simulink library "Lib_Vol_PropLookup_TMATS"  (R2015a)
settings: Solver=ode45  StartTime=0.0  StopTime=10.0  RelTol=1e-3
undefined symbols (not defined in the file or in its folder): hP_PropArray_M, htVec_M, PtVec_M, sP_PropArray_M, sVec_M, TtVec_M
Description:
  | Thomas Modules
settings Model: Creator=jwchapm2  LastModifiedBy=jwchapm2
settings OptimizationCC: ExpressionDepthLimit=2147483647
settings DebuggingCC: UnderspecifiedInitializationDetection=Classic  MergeDetectMultiDrivingBlocksExec=none  SolverPrmCheckMsg=warning  StateNameClashWarn=warning

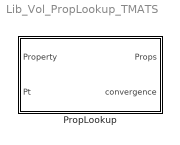
== system Lib_Vol_PropLookup_TMATS ==
  PropLookup : Subsystem  TreatAsAtomicUnit=on  mask(T-MATS: PropLookup Library Block){case_M='ht', propg_M=0, htg_M=0, htVec_M=[0 10], PtVec_M=[0 10], TtVec_M=[0 10], sVec_M=[0 10], htArray_M=ones(length(TtVec_M), length(PtVec_M)), rhoArray_M=ones(length(htVec_M), length(PtVec_M)), uArray_M=ones(length(htVec_M), length(PtVec_M)), sArray_M=ones(length(htVec_M), length(PtVec_M)), muArray_M=ones(length(htVec_M), length(PtVec_M)), ThArray_M=ones(length(htVec_M), length(PtVec_M)), CvArray_M=ones(length(htVec_M), length(PtVec_M)), CpArray_M=ones(length(htVec_M), length(PtVec_M)), kArray_M=ones(length(htVec_M), length(PtVec_M)), TsArray_M=ones(length(sVec_M), length(PtVec_M)), hsArray_M=ones(length(sVec_M), length(PtVec_M)), Rval_M=0}
      mask prompts: case_M "case_M - Property type"; propg_M "propg_M - Initial guess for property value"; htg_M "htg_M - Initial guess for ethanply value"; htVec_M "htVec_M - ht axis for table lookup"; PtVec_M "PtVec_M - Pt axis for table lookup"; TtVec_M "TtVec_M - Tt axis for table lookup"; sVec_M "sVec_M - s axis for table lookup"; htArray_M "htArray_M - enthlapy Array f(Tt,Pt)"; rhoArray_M "rhoArray_M - rho Array f(ht,Pt)"; uArray_M "uArray_M - u Array f(ht,Pt)"; sArray_M "sArray_M - s Array f(ht,Pt)"; muArray_M "muArray_M - mu Array f(ht,Pt)"; ThArray_M "ThArray_M - Th Array f(ht,Pt)"; CvArray_M "CvArray_M - Cv Array f(ht,Pt)"; CpArray_M "CpArray_M - Cp Array f(ht,Pt)"; kArray_M "kArray_M - k Array f(ht,Pt)"; TsArray_M "TsArray_M - Ts Array f(s,Pt)"; hsArray_M "hsArray_M - hs Array f(s,Pt)"; Rval_M "Rval_M - R value"
      mask help: This block is used to model the thermodynamic properties of a mass flow based on table lookups.
      mask init:
      | hP_PropArray_M(:,:,1) = rhoArray_M;
      | hP_PropArray_M(:,:,2) = uArray_M;
      | hP_PropArray_M(:,:,3) = sArray_M;
      | hP_PropArray_M(:,:,4) = muArray_M;
      | hP_PropArray_M(:,:,5) = ThArray_M;
      | hP_PropArray_M(:,:,6) = CvArray_M;
      | hP_PropArray_M(:,:,7) = kArray_M;
      | hP_PropArray_M(:,:,8) = CpArray_M;
      | 
      | sP_PropArray_M(:,:,1) = TsArray_M;
      | sP_PropArray_M(:,:,2) = hsArray_M;
      | 
      | case_M = double(case_M);
      mask Help: web(which('Vol_TMATS_PropLookup.html'),'-helpbrowser')

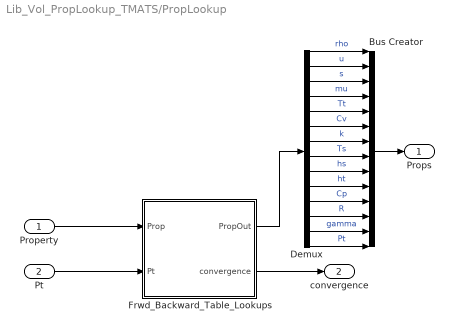
== system Lib_Vol_PropLookup_TMATS/PropLookup ==
  Property : Inport
  Pt : Inport  Port=2
  Bus Creator : BusCreator  Inputs=14
  Demux : Demux  Outputs=14
  Frwd_Backward_Table_Lookups : MATLAB Function  TreatAsAtomicUnit=on
  Props : Outport
  convergence : Outport  Port=2
  wires:
  Property/1 -> Frwd_Backward_Table_Lookups/1(Prop)
  Pt/1 -> Frwd_Backward_Table_Lookups/2(Pt)
  Frwd_Backward_Table_Lookups/2(convergence) -> convergence/1
  Demux/13 -> Bus Creator/13  "gamma"
  Demux/12 -> Bus Creator/12  "R"
  Demux/11 -> Bus Creator/11  "Cp"
  Demux/10 -> Bus Creator/10  "ht"
  Demux/8 -> Bus Creator/8  "Ts"
  Demux/7 -> Bus Creator/7  "k"
  Demux/4 -> Bus Creator/4  "mu"
  Demux/9 -> Bus Creator/9  "hs"
  Demux/6 -> Bus Creator/6  "Cv"
  Demux/3 -> Bus Creator/3  "s"
  Demux/5 -> Bus Creator/5  "Tt"
  Demux/2 -> Bus Creator/2  "u"
  Demux/1 -> Bus Creator/1  "rho"
  Bus Creator/1 -> Props/1
  Frwd_Backward_Table_Lookups/1(PropOut) -> Demux/1
  Demux/14 -> Bus Creator/14  "Pt"

== matlab function Lib_Vol_PropLookup_TMATS/PropLookup/Frwd_Backward_Table_Lookups ==
  data: Prop input; Pt input; PropOut output; convergence output; htg_M parameter; htVec_M parameter; TtVec_M parameter; PtVec_M parameter; sVec_M parameter; htArray_M parameter; hP_PropArray_M parameter; sP_PropArray_M parameter; Rval_M parameter; case_M parameter
function [PropOut, convergence] = fcn(Prop, Pt, htg_M, htVec_M, TtVec_M, PtVec_M, sVec_M, htArray_M, hP_PropArray_M, sP_PropArray_M, Rval_M, case_M)
% Table lookup based on ht or ht guess

%gather table vector table data
htVec = htVec_M;
TtVec = TtVec_M;
PtVec = PtVec_M;
sVec = sVec_M;

% determine min and max table lookup values
Tmx = max(TtVec);
Tmn = min(TtVec);
hmx = max(htVec);
hmn = min(htVec);
Pmx = max(PtVec);
Pmn = min(PtVec);
smx = max(sVec);
smn = min(sVec);

Pt_tbl = max(min(Pt,Pmx),Pmn);

%gather table array data
rhoArray    =  hP_PropArray_M(:,:,1);
uArray      =  hP_PropArray_M(:,:,2);
sArray      =  hP_PropArray_M(:,:,3);
muArray     =  hP_PropArray_M(:,:,4);
ThArray     =  hP_PropArray_M(:,:,5);
CvArray     =  hP_PropArray_M(:,:,6);
kArray      =  hP_PropArray_M(:,:,7);
CpArray     =  hP_PropArray_M(:,:,8);


TsArray = sP_PropArray_M(:,:,1);
hsArray = sP_PropArray_M(:,:,2);

htArray = htArray_M;


switch char(case_M)
    case 'ht'
        iterate = 0;
        htg = Prop;
    case 'Tt'
        iterate = 0;
        T_tbl = max(min(Prop,Tmx),Tmn);
        htg = interp2(TtVec, PtVec, htArray,T_tbl, Pt_tbl);
    otherwise
        iterate = 1;
end

iter = 0;
maxiter = 15 ;

if iterate == 1 % ht is unknown,  iterate to find it based on what Prop is
    
    % determine initial error, ht guess term, and iteration constants
    switch char(case_M)
        case 'u'
            itprop = interp2(htVec, PtVec, rhoArray,htg_M, Pt);
        case 's'
            itprop = interp2(htVec, PtVec, sArray,htg_M, Pt);
        case 'k'
            itprop = interp2(htVec, PtVec, kArray,htg_M, Pt);
        case 'Ts'
            s_prop = interp2(htVec, PtVec, sArray,htg_M, Pt);
            itprop = interp2(sVec, PtVec, TsArray,s_prop, Pt);
        case 'hs'
            s_prop = interp2(htVec, PtVec, sArray,htg_M, Pt);
            itprop = interp2(sVec, PtVec, hsArray, s_prop, Pt);
        otherwise
            itprop = 0;
    end
    Error = Prop - itprop;
    htg_new = htg_M + 0.002;
    erthr = 0.0001;
    htg = htg_M;
    
    while ((abs(Error) > erthr) && (iter < maxiter))
        % Set old values before recaulcation
        Er_old = Error;
        htg_old = htg;
        
        % if step is too low assume larger step
        if abs(htg - htg_new) < 0.001
            htg = htg + 0.002;
        else
            htg = htg_new;
        end
        
        htg_tbl = max(min(htg,hmx),hmn);
        
        % Determine property term based on guessed ht
        switch char(case_M)
            case 'u'
                itprop = interp2(htVec, PtVec, rhoArray,htg_tbl, Pt_tbl);
            case 's'
                itprop = interp2(htVec, PtVec, sArray,htg_tbl, Pt_tbl);
            case 'k'
                itprop = interp2(htVec, PtVec, kArray,htg_tbl, Pt_tbl);
            case 'Ts'
                s_prop = interp2(htVec, PtVec, sArray,htg_tbl, Pt_tbl);
                s_ptbl = max(min(s_prop,smx),smn);
                itprop = interp2(sVec, PtVec, TsArray,s_ptbl, Pt_tbl);
            case 'hs'
                s_prop = interp2(htVec, PtVec, sArray,htg_tbl, Pt_tbl);
                s_ptbl = max(min(s_prop,smx),smn);
                itprop = interp2(sVec, PtVec, hsArray, s_ptbl, Pt_tbl);
            otherwise
                itprop = 0;
        end
        % determine current property term error
        Error = Prop - itprop;
        
        if (abs(Error) > erthr)
            % determine new guess enthalpy by secant algorithm
            htg_new = htg - Error *(htg - htg_old)/(Error - Er_old);
        end
        iter = iter +1;
    end
end

if iter >= maxiter
    convergence = 0;
else
    convergence = 1;
end

%generate outputs based on ht (found by input, table lookup, or iteration)
ht = htg;

ht_tbl = max(min(ht,hmx),hmn);

% ht, Pt generated lookups
rho = interp2(htVec, PtVec, rhoArray,ht_tbl, Pt_tbl);
u =  interp2(htVec, PtVec, uArray,ht_tbl, Pt_tbl);
s = interp2(htVec, PtVec, sArray,ht_tbl, Pt_tbl);
mu = interp2(htVec, PtVec, muArray,ht_tbl, Pt_tbl);
Th = interp2(htVec, PtVec, ThArray,ht_tbl, Pt_tbl);
Cv = interp2(htVec, PtVec, CvArray,ht_tbl, Pt_tbl);
k = interp2(htVec, PtVec, kArray,ht_tbl, Pt_tbl);
Cp = interp2(htVec, PtVec, CpArray, ht_tbl, Pt_tbl);


% s, Pt generated lookups
s_tbl = max(min(s,smx),smn);
Ts = interp2(sVec, PtVec, TsArray, s_tbl, Pt_tbl);
hs = interp2(sVec, PtVec, hsArray, s_tbl, Pt_tbl);
% Other lookups
R = Rval_M;
gamma = Cp/Cv;


PropOut = [rho u s mu Th Cv k Ts hs ht Cp R gamma Pt]';
